simulink model "untitled3"  (R2023b)
settings: Solver=VariableStepAuto  StartTime=0.0  StopTime=10.0  RelTol=1e-3
libraries: checkpacklib x2
settings Model: Creator=a2  LastModifiedBy=a2
settings DataIOCC: ReturnWorkspaceOutputsName=SDOSimTest_Log

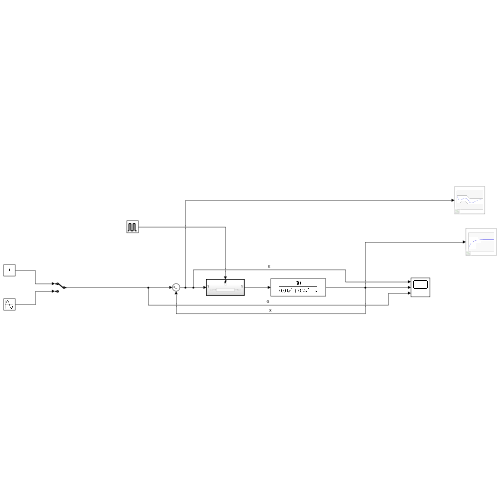
[thumbnail: Simulink's stored preview of the top-level diagram]
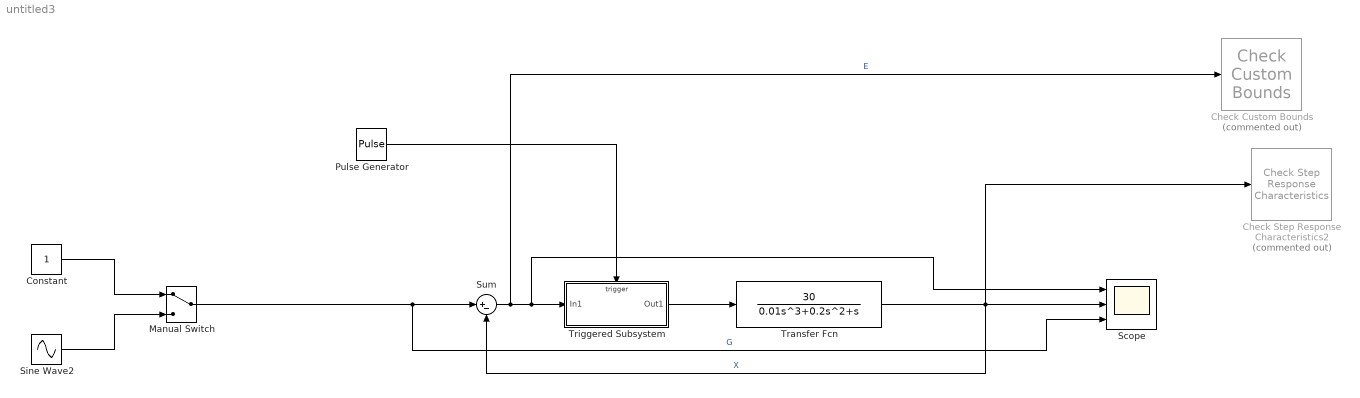
== system untitled3 ==
  Check Custom Bounds : checkpacklib/Check Custom Bounds  Commented=on  InstantiateOnLoad=on  enabled=on  stopWhenAssertionFail=off  export=off  ViewDlgPos=[]  OpenViewOnLoad=off  LaunchViewOnOpen=off  TimeUnits=seconds  EnableUpperBound=on  UpperBoundTimes=[0 5; 5 10]  UpperBoundAmplitudes=[5 5; 1 1]  EnableLowerBound=on  LowerBoundTimes=[0 5; 5 10]  LowerBoundAmplitudes=[-5 -5; -1 -1]
      settings: LibrarySourceBlock=sdolib/Model Verification/Check Custom Bounds
  Check Step Response Characteristics2 : checkpacklib/Check Step Response  Characteristics  Commented=on  InstantiateOnLoad=on  enabled=on  stopWhenAssertionFail=off  export=off  ViewDlgPos=[]  OpenViewOnLoad=off  LaunchViewOnOpen=off  TimeUnits=seconds  EnableStepResponseBound=on  InitialValue=0  FinalValue=1  StepTime=0  RiseTime=5  PercentRise=80  SettlingTime=7  PercentSettling=1  PercentOvershoot=10  PercentUndershoot=1
      settings: LibrarySourceBlock=|
      | sdolib/Model Verification/Check Step Response
      | Characteristics
  Constant : Constant
  Manual Switch : ManualSwitch
  Pulse Generator : DiscretePulseGenerator  PulseType=Time based  Period=0.005  PulseWidth=5
  Scope : Scope  NumInputPorts=3
  Sine Wave2 : Sin  Amplitude=50  Frequency=0.5  SampleTime=0
  Sum : Sum  Inputs=|+-
  Transfer Fcn : TransferFcn  Numerator=[30]  Denominator=[0.01 0.2 1 0]
  Triggered Subsystem : Subsystem  TreatAsAtomicUnit=on
  wires:
  Sum/1 -> Check Custom Bounds/1, Scope/1, Triggered Subsystem/1(In1)  "E"
  Transfer Fcn/1 -> Sum/2, Scope/2, Check Step Response Characteristics2/1  "X"
  Manual Switch/1 -> Scope/3, Sum/1  "G"
  Pulse Generator/1 -> Triggered Subsystem/Trigger
  Triggered Subsystem/1(Out1) -> Transfer Fcn/1
  Sine Wave2/1 -> Manual Switch/2
  Constant/1 -> Manual Switch/1

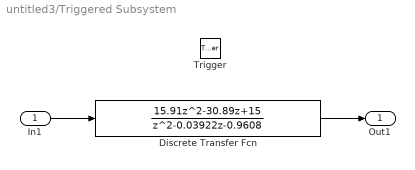
== system untitled3/Triggered Subsystem ==
  In1 : Inport
  Trigger : TriggerPort  VariantControl=(inherit)
  Discrete Transfer Fcn : DiscreteTransferFcn  Numerator=[15.91 -30.89 15]  Denominator=[1 -0.03922 -0.9608]
  Out1 : Outport
  wires:
  Discrete Transfer Fcn/1 -> Out1/1
  In1/1 -> Discrete Transfer Fcn/1
